simulink model "hand_exo"  (R2016a)
settings: Solver=ode15s  StartTime=0.0  StopTime=15  RelTol=1e-8
settings Model: Creator=FPCC  LastModifiedBy=FPCC
settings SolverCC: ZeroCrossControl=DisableAll  ZeroCrossAlgorithm=Adaptive

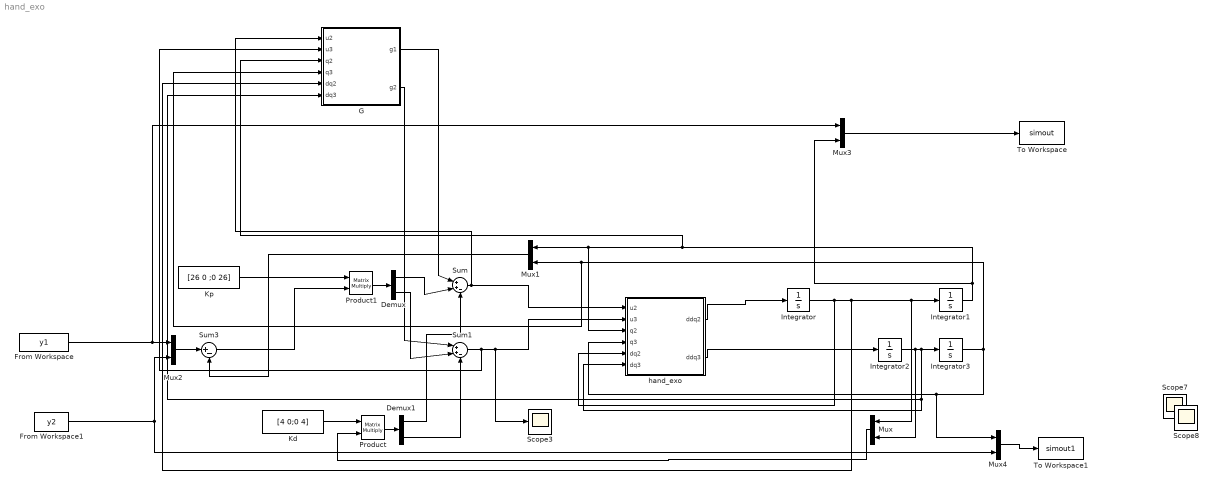
== system hand_exo ==
  Demux : Demux  Outputs=2
  Demux1 : Demux  Outputs=2
  From Workspace : FromWorkspace  VariableName=y1  SampleTime=0
  From Workspace1 : FromWorkspace  VariableName=y2  SampleTime=0
  G : MATLAB Function  TreatAsAtomicUnit=on
  Integrator : Integrator  UpperSaturationLimit=10  LowerSaturationLimit=-10  IgnoreLimit=on  ZeroCross=off
  Integrator1 : Integrator  UpperSaturationLimit=100  LowerSaturationLimit=-100
  Integrator2 : Integrator  UpperSaturationLimit=100  LowerSaturationLimit=-100
  Integrator3 : Integrator  UpperSaturationLimit=100  LowerSaturationLimit=-100
  Kd : Constant  Value=[4 0;0 4]
  Kp : Constant  Value=[26 0 ;0 26]
  Mux{,1..4} (5 alike) : Mux  Inputs=2
  Product : Product  Multiplication=Matrix(*)
  Product1 : Product  Multiplication=Matrix(*)
  Scope3 : Scope
  Scope7 : Scope
  Scope8 : Scope
  Sum : Sum  Inputs=|++-
  Sum1 : Sum  Inputs=|++-
  Sum3 : Sum  Inputs=|+-
  To Workspace : ToWorkspace  VariableName=simout  SaveFormat=Timeseries  SampleTime=-1
  To Workspace1 : ToWorkspace  VariableName=simout1  SaveFormat=Timeseries  SampleTime=-1
  hand_exo : MATLAB Function  TreatAsAtomicUnit=on
  wires:
  Integrator/1 -> hand_exo/5(dq2), G/5(dq2), Mux/1, Integrator1/1
  Integrator2/1 -> Mux/2, G/6(dq3), hand_exo/6(dq3), Integrator3/1
  Kp/1 -> Product1/1
  Kd/1 -> Product/1
  Mux/1 -> Product/2
  Product1/1 -> Demux/1
  Product/1 -> Demux1/1
  Demux/1 -> Sum/2
  Demux/2 -> Sum1/2
  Demux1/1 -> Sum/3
  Demux1/2 -> Sum1/3
  hand_exo/2(ddq3) -> Integrator2/1
  Mux2/1 -> Sum3/1
  Sum3/1 -> Product1/2
  Sum1/1 -> G/2(u3), Scope3/1, hand_exo/2(u3)
  Integrator1/1 -> G/3(q2), hand_exo/3(q2), Mux1/1, Mux3/2
  Mux3/1 -> To Workspace/1
  hand_exo/1(ddq2) -> Integrator/1
  Integrator3/1 -> G/4(q3), Mux1/2, Mux4/1, hand_exo/4(q3)
  From Workspace1/1 -> Mux2/2, Mux4/2
  Mux4/1 -> To Workspace1/1
  Mux1/1 -> Sum3/2
  Sum/1 -> hand_exo/1(u2), G/1(u2)
  G/1(g1) -> Sum/1
  G/2(g2) -> Sum1/1
  From Workspace/1 -> Mux3/1, Mux2/1

== matlab function hand_exo/G ==
  data: u2 input; g1 output; u3 input; q2 input; q3 input; dq2 input; dq3 input; g2 output
function [g1,g2]  = fcn(u2,u3,q2,q3,dq2,dq3)
% L1 = 12; L2 = 20; L3 = 45; L4 = 15; L5 = 20;
% m1 = 100; m2 = 70; m3 = 170; m4 = 100; m5 = 20;
% I1 = m1*L1^2/3; I2 = m2*L2^2/3; I3 = m3*L3^2/3; I4 =m4*L4^2/3; I5 = m5*L5^2/3;
% V=47;
% H=20;


L1 = 12/1000; L2 = 20/1000; L3 = 45/1000; L4 = 15/1000; L5 = 20/1000;
m1 = 100/1000; m2 = 70/1000; m3 = 170/1000; m4 = 100/1000; m5 = 20/1000;
I1 = m1*L1^2/3; I2 = m2*L2^2/3; I3 = m3*L3^2/3; I4 =m4*L4^2/3; I5 = m5*L5^2/3;

V=47/1000;
H=20/1000;


q1 = (L1 - V) * tan(q2);

q4=q3;
dq4=dq3;

q5=((H-L4*cos(q3+q4)-L3*cos(q3))/cos(q3+q4));
dq5=((L3*sin(q3)*dq3*cos(q3+q4)+sin(q3+q4)*(dq3+dq4)*(H-L3*cos(q3)))/cos(q3+q4)^2);




% Inertia matrices (placeholders, replace with actual inertia tensors)
%

% Gravitational acceleration
g = 9.82;

G=[0;
 g*cos(q3)*(L2*m3 + L2*m4 + L2*m5 + L3*m4*cos(q4) + L3*m5*cos(q4) + L4*m5*cos(q4))];
g1=G(1);
g2=G(2);

== matlab function hand_exo/hand_exo ==
  data: u2 input; ddq2 output; u3 input; ddq3 output; q2 input; q3 input; dq2 input; dq3 input
function [ddq2,ddq3] = fcn(u2,u3,q2,q3,dq2,dq3)
% L1 = 12; L2 = 20; L3 = 45; L4 = 15; L5 = 20;
% m1 = 100; m2 = 70; m3 = 170; m4 = 100; m5 = 20;
% I1 = m1*L1^2/3; I2 = m2*L2^2/3; I3 = m3*L3^2/3; I4 =m4*L4^2/3; I5 = m5*L5^2/3;
% V=47;
% H=20;


L1 = 12/1000; L2 = 20/1000; L3 = 45/1000; L4 = 15/1000; L5 = 20/1000;
m1 = 100/1000; m2 = 70/1000; m3 = 170/1000; m4 = 100/1000; m5 = 20/1000;
I1 = m1*L1^2/3; I2 = m2*L2^2/3; I3 = m3*L3^2/3; I4 =m4*L4^2/3; I5 = m5*L5^2/3;

V=47/1000;
H=20/1000;


q1 = (L1 - V) * tan(q2);
% A = V - L1 - (L2 + L3*cos(q3)) * cos(q2);
% B = (H - L3*sin(q3)) * cos(q2);
% C = L4 * cos(q2);
% R = sqrt(A^2 + B^2-C^2);
% phi = atan2(A, B);
% 
% 
% dA=L2*sin(q2)*dq2-L3*(sin(q3)*cos(q2)*dq3+cos(q3)*sin(q2)*dq2);
% dB=L3*(sin(q3)*sin(q2)*dq2-cos(q3)*cos(q2)*dq3)-H*sin(q2)*dq2;
% dC=-L4*sin(q2)*dq2;
% 
% dR=(A*dA+dB*B-C*dC)/R;
% dphi=(dA*B-dB*A)/(B^2)/(1+(A/B)^2);
% 
% 
% 
% qtemp1 = atan2(C , R) - phi;
% %qtemp2 = -acos(C / R) + phi;
% q4 = qtemp1 - q3;
% dq4=(C*dR-dC*R)/(R^2)/(1+(C/R)^2)+ dphi - dq3;
q4=q3;
dq4=dq3;

q5=((H-L4*cos(q3+q4)-L3*cos(q3))/cos(q3+q4));
dq5=((L3*sin(q3)*dq3*cos(q3+q4)+sin(q3+q4)*(dq3+dq4)*(H-L3*cos(q3)))/cos(q3+q4)^2);




% Inertia matrices (placeholders, replace with actual inertia tensors)
%

% Gravitational acceleration
g = 9.82;
J=[1e-6 0;0 1e-6 ];
M=[m2*L1^2-I2*cos(q2) 0;
    0 L2^2*m3-I3*cos(q3)+I3*cos(q2)^2+I3*cos(q2)^2*cos(q3)];
invM=inv(M);
C=[ (I2*dq2^2*sin(q2))/2 + (I3*dq3^2*sin(2*q2))/2 - (I5*dq5^2*sin(2*q2))/2 - (I4*dq4^2*cos(q2)*sin(q4))/2 - (I4*dq4^2*cos(q4)*sin(q2))/2 + (I4*dq4^2*cos(q2)*cos(q3)^2*sin(q4))/2 + (I4*dq4^2*cos(q3)^2*cos(q4)*sin(q2))/2 + I5*dq5^2*cos(q2)*cos(q3)^2*sin(q2) - (I5*dq5^2*cos(q2)*cos(q3)^2*sin(q4))/2 + I3*dq3^2*cos(q2)*cos(q3)*sin(q2) - (I5*dq5^2*cos(q3)*cos(q4)*sin(q2))/2 - (I5*dq5^2*cos(q3)*cos(q4)*sin(q3))/2 + I5*dq5^2*cos(q2)^2*cos(q3)*cos(q4)*sin(q3) - I5*dq5^2*cos(q2)*sin(q2)*sin(q3)*sin(q4);
 (I3*dq3^2*sin(q3))/2 + (I4*dq4^2*sin(2*q3))/2 - (I5*dq5^2*sin(2*q3))/2 - (I3*dq3^2*cos(q2)^2*sin(q3))/2 - I3*dq2*dq3*sin(2*q2) + I5*dq5^2*cos(q2)^2*cos(q3)*sin(q3) + (I5*dq5^2*cos(q2)^2*cos(q3)*sin(q4))/2 - (I5*dq5^2*cos(q2)*cos(q4)*sin(q2))/2 - (I5*dq5^2*cos(q2)*cos(q4)*sin(q3))/2 + I5*dq5^2*cos(q2)*cos(q3)^2*cos(q4)*sin(q2) + I4*dq4^2*cos(q2)*cos(q3)*cos(q4)*sin(q3) - I4*dq4^2*cos(q3)*sin(q2)*sin(q3)*sin(q4) + I5*dq5^2*cos(q3)*sin(q2)*sin(q3)*sin(q4) - 2*I3*dq2*dq3*cos(q2)*cos(q3)*sin(q2)];
G=[0;0];
M=M+J;
G=[0;
 g*cos(q3)*(L2*m3 + L2*m4 + L2*m5 + L3*m4*cos(q4) + L3*m5*cos(q4) + L4*m5*cos(q4))];
ddq=[0;0];
ddq=invM*([u2;u3]-C-G);
ddq2=ddq(1);
ddq3=ddq(2);
